simulink model "EmbeddedControl"  (R2022a)
settings: Solver=FixedStepDiscrete  StartTime=0.0  StopTime=inf  FixedStep=0.02  RelTol=1e-3  EnableMultiTasking=on
model workspace (MAT data in the model file):
  Ts = 0.02
libraries: instrumentseriallib x3
settings Model: Creator=Rafael  LastModifiedBy=Rafael
settings SolverCC: ConcurrentTasks=on  PositivePriorityOrder=on
settings OptimizationCC: BlockReduction=off  EnhancedBackFolding=on  PassReuseOutputArgsAs=Individual arguments  ZeroExternalMemoryAtStartup=off  ZeroInternalMemoryAtStartup=off  MaxStackSize=64  OptimizeBlockOrder=speed  DifferentSizesBufferReuse=on  OptimizationCustomize=off  EfficientTunableParamExpr=on
settings DebuggingCC: TasksWithSamePriorityMsg=none  ParameterTunabilityLossMsg=error
settings HardwareCC: ProdBitPerPointer=32  ProdBitPerSizeT=32  ProdBitPerPtrDiffT=32  ProdLargestAtomicInteger=Long  ProdLargestAtomicFloat=Double  ProdWordSize=32  ProdLongLongMode=on  ProdHWDeviceType=ARM Compatible->ARM Cortex  TargetBitPerPointer=64  TargetBitPerSizeT=64  TargetBitPerPtrDiffT=64  TargetLongLongMode=on  TargetIntDivRoundTo=Zero  TargetEndianess=LittleEndian  TargetWordSize=64  TargetHWDeviceType=MATLAB Host
settings SFSimCC: MATLABDynamicMemAlloc=off
settings RTWCC: SystemTargetFile=ert.tlc  HardwareBoard=STM32F4xx Based  TemplateMakefile=ert_default_tmf  Toolchain=GNU Tools for ARM Embedded Processors  BuildConfiguration=Faster Runs  CodeExecutionProfiling=on  TargetLang=C++
settings CodeAppCC: ForceParamTrailComments=on  IgnoreCustomStorageClasses=off  MaxIdLength=95  OperatorAnnotations=on  SimulinkDataObjDesc=on  SFDataObjDesc=on  InsertBlockDesc=on
settings ERTTargetCC: CodeReplacementLibrary=ARM Cortex-M  ExtModeTransport=3  ExtModeStaticAlloc=on  ExtModeStaticAllocSize=2048  ExtModeMexFile=ext_xcp  ExtModeIntrfLevel=Level2 - Open  RootIOFormat=Structure reference

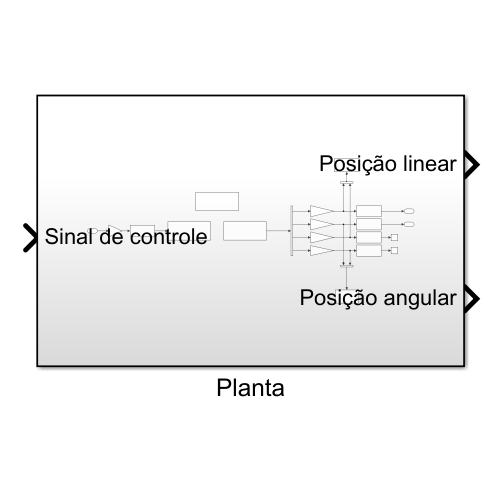
[thumbnail: Simulink's stored preview of the top-level diagram]
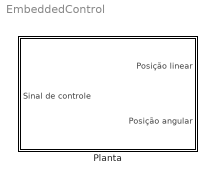
== system EmbeddedControl ==
  Planta : Subsystem

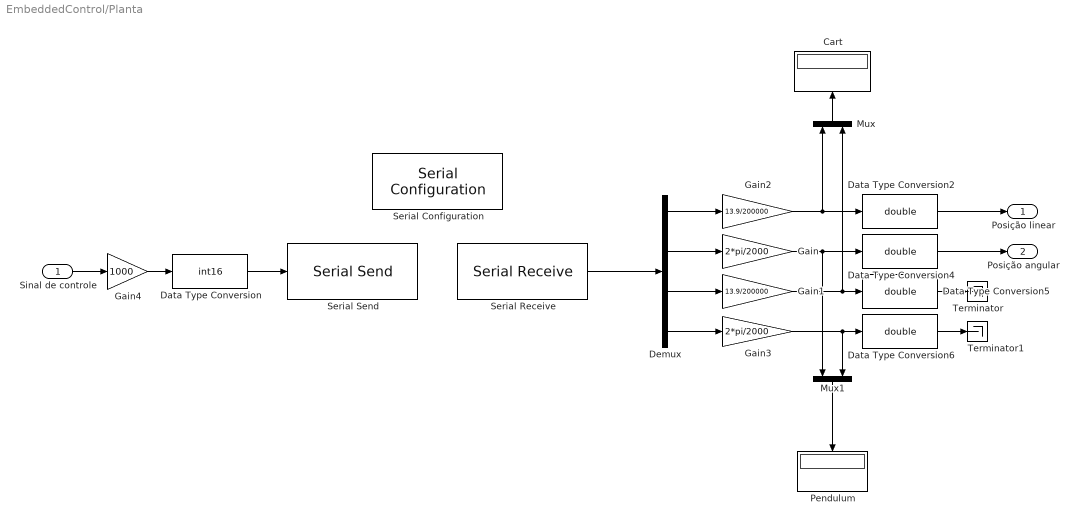
== system EmbeddedControl/Planta ==
  Sinal de controle : Inport
  Cart : Display
  Data Type Conversion : DataTypeConversion  OutMin=[-1000]  OutMax=[1000]  OutDataTypeStr=int16  SaturateOnIntegerOverflow=off  RndMeth=Floor
  Data Type Conversion{2,4..6} (4 alike) : DataTypeConversion  OutMin=[-65000]  OutMax=[65000]  OutDataTypeStr=double  SaturateOnIntegerOverflow=off  RndMeth=Floor
  Demux : Demux
  Gain : Gain  Gain=2*pi/2000
  Gain1 : Gain  Gain=13.9/200000
  Gain2 : Gain  Gain=13.9/200000
  Gain3 : Gain  Gain=2*pi/2000
  Gain4 : Gain  Gain=1000
  Mux : Mux  Inputs=2
  Mux1 : Mux  Inputs=2
  Pendulum : Display
  Serial Configuration : instrumentseriallib/Serial Configuration  Priority=-200000  PortSel=COM9  Port=COM9  ComPort=COM9  BaudRate=115200  DataBits=8  Parity=none  StopBits=1  ByteOrder=little-endian  FlowControl=none  Timeout=10  SimulateUsing=Interpreted execution  BlockInModel=on  aMode=1
      settings: SourceProductBaseCode=OT,IC,MT
  Serial Receive : instrumentseriallib/Serial Receive  Priority=1  PortSel=COM9  Port=COM9  ComPort=COM9  DataType=int16  SaveDataType=uint8  ToggleHeader=on  Header=[35]  ToggleTerminator=on  Terminator=<none>  CustomTerminator=[]  InputFormat=Column major  ToggleDataSize=on  DataSize=[1 4]  EnableBlockingMode=on  ActionDataUnavailable=Output last received value  ActionWhenDataUnavailable=Output last received value  CustomValue=0  SampleTime=-1  SimulateUsing=Interpreted execution  BlockInModel=on  aMode=1
      settings: SourceProductBaseCode=OT,IC,MT
  Serial Send : instrumentseriallib/Serial Send  Priority=1  PortSel=COM9  Port=COM9  ComPort=COM9  Header=[]  Terminator=<none>  CustomTerminator=[]  EnableBlockingMode=off  SimulateUsing=Interpreted execution  BlockInModel=on  aMode=1
      settings: SourceProductBaseCode=OT,IC,MT
  Terminator : Terminator
  Terminator1 : Terminator
  Posição linear : Outport
  Posição angular : Outport  Port=2
  wires:
  Serial Receive/1 -> Demux/1
  Mux/1 -> Cart/1
  Gain1/1 -> Data Type Conversion5/1, Mux/2
  Demux/4 -> Gain3/1
  Gain2/1 -> Data Type Conversion2/1, Mux/1
  Gain3/1 -> Data Type Conversion6/1, Mux1/2
  Demux/3 -> Gain1/1
  Demux/1 -> Gain2/1
  Gain/1 -> Data Type Conversion4/1, Mux1/1
  Mux1/1 -> Pendulum/1
  Demux/2 -> Gain/1
  Data Type Conversion2/1 -> Posição linear/1
  Data Type Conversion4/1 -> Posição angular/1
  Sinal de controle/1 -> Gain4/1
  Data Type Conversion5/1 -> Terminator/1
  Data Type Conversion6/1 -> Terminator1/1
  Gain4/1 -> Data Type Conversion/1
  Data Type Conversion/1 -> Serial Send/1
